simulink model "EVCS_model_v2"  (R2024b)
settings: Solver=VariableStepAuto  StartTime=0.0  StopTime=210  MaxStep=1e-3  RelTol=1e-2  AbsTol=1e-3
undefined symbols (not defined in the file or in its folder): FC, gcbh, Ion, Lithium, P, sps_rtmsupport, Ts
libraries: spsSeriesRLCBranchLib x40, spsIGBTDiodeLib x8, slpidlib x7, spsVoltageMeasurementLib x7, spsCurrentMeasurementLib x6, eeGeneralControl x4, spsMosfetLib x4, spsPWMGeneratorDCDCLib x3, spsAlphaBetaZerotodq0Lib x2, spsBatteryLib x2, spsDiodeLib x2, spsBreakerLib x1
(part 2 of 2)

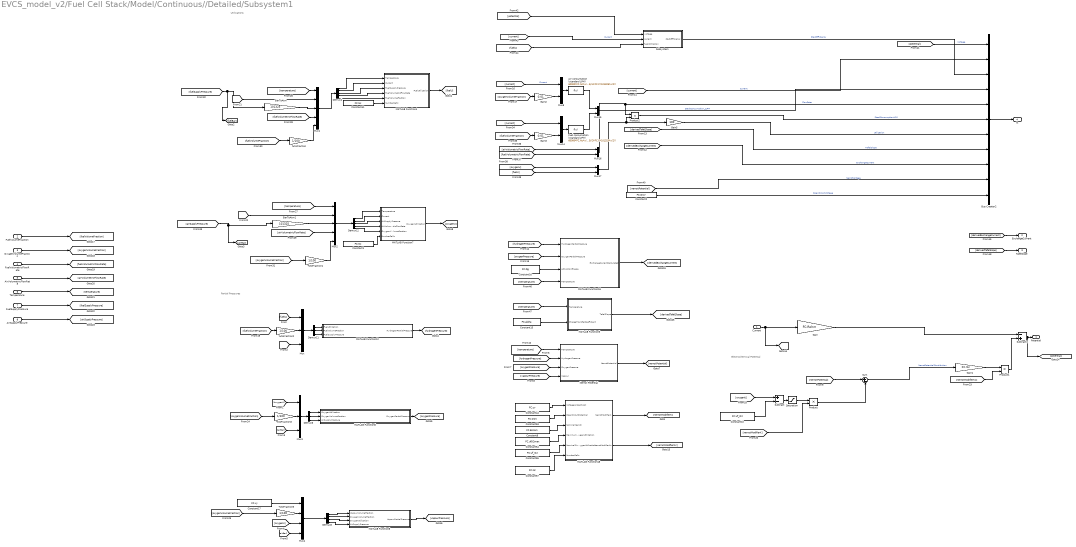
== system EVCS_model_v2/Fuel Cell Stack/Model/Continuous//Detailed/Subsystem1 ==
  note: Electrochemical Potential
  note: Partial Pressures
  note: Utilizations
  Current : Inport
  FuelVolumeFraction : Inport  Port=2
  OxygenVolumeFraction : Inport  Port=3
  FuelVolumetricFlowRate : Inport  Port=4
  AirVolumetricFlowRate : Inport  Port=5
  Temperature : Inport  Port=6
  FuelSupplyPressure : Inport  Port=7
  AirSupplyPressure : Inport  Port=8
  %toFraction{,1..3,5} (5 alike) : Gain  Gain=1/100
  Air consumption (standard LPM) : Fcn  Expr=60000*FC.Nc*u(1)*FC.R*293.15/(4*FC.F*101325*u(2))
  BarToAtm : Gain  Gain=101325
  BarToAtm1 : Gain  Gain=101325
  Bus Creator2 : BusCreator  Inputs=11
  Constant1 : Constant  Value=FC.Nc
  Constant10 : Constant  Value=FC.Uf_O2
  Constant15 : Constant  Value=FC.alpha
  Constant16 : Constant  Value=FC.Dg
  Constant17 : Constant  Value=FC.xy
  Constant2 : Constant  Value=FC.OCV
  Constant41 : Constant  Value=FC.Nc
  Constant44 : Constant  Value=FC.uv
  Constant53 : Constant  Value=FC.OCV
  Constant54 : Constant  Value=FC.ufO2max
  Constant55 : Constant  Value=FC.Uf_O2
  Constant57 : Constant  Value=FC.Nc
  Constant8 : Constant  Value=FC.Ennom
  Demux11 : Demux  Outputs=3
  Demux12 : Demux  Outputs=5
  Demux4 : Demux  Outputs=5
  Demux6 : Demux  Outputs=3
  Demux8 : Demux
  Fuel consumption (standard LPM) : Fcn  Expr=60000*FC.Nc*u(1)*FC.R*293.15/(2*FC.F*101325*u(2))
  Gain : Gain  Gain=FC.Rohm
  Gain1 : Gain  Gain=FC.Nc
  Gain2 : Gain  Gain=0.01
  Gain3 : Gain  Gain=0.01
  Gain5 : Gain  Gain=100
  MATLAB Function12 : MATLAB Function  TreatAsAtomicUnit=on
  MATLAB Function16 : MATLAB Function  TreatAsAtomicUnit=on
  MATLAB Function18 : MATLAB Function  TreatAsAtomicUnit=on
  MATLAB Function4 : MATLAB Function  TreatAsAtomicUnit=on
  MATLAB Function5 : MATLAB Function  TreatAsAtomicUnit=on
  MATLAB Function6 : MATLAB Function  TreatAsAtomicUnit=on
  MATLAB Function7 : MATLAB Function  TreatAsAtomicUnit=on
  MATLAB Function8 : MATLAB Function  TreatAsAtomicUnit=on
  Mux : Mux  Inputs=3
  Mux1 : Mux  Inputs=5
  Mux{8,14..17} (5 alike) : Mux  Inputs=2
  Mux2 : Mux  Inputs=5
  Mux3 : Mux  Inputs=3
  Mux4 : Mux
  Nernst Potential : Subsystem
  Product : Product
  Product1 : Product
  Product2 : Product  RndMeth=Zero
  Saturation : Saturate  UpperLimit=inf  LowerLimit=0
  Subsystem : Subsystem
  Subtract : Sum  Inputs=+-
  Subtract1 : Sum  Inputs=-+
  Sum : Sum  Inputs=|+-
  Potential : Outport
  ExchangeCurrent : Outport  Port=2
  TafelSlope : Outport  Port=3
  m : Outport  Port=4
  wires:
  %toFraction3/1 -> Mux3/2
  Constant2/1 -> Bus Creator2/11  "OpenCircuitVoltage"
  Demux4/4 -> MATLAB Function4/4(FuelVolumetricFlowRate)
  [temperature] -> MATLAB Function16/4(Temperature)
  [oxygenU] -> Mux3/1
  Demux4/1 -> MATLAB Function4/1(Temperature)
  AirSupplyPressure/1 -> [airSupplyPressure]
  [fuelVolumeFraction] -> Gain3/1
  BarToAtm1/1 -> Mux2/3
  Constant55/1 -> MATLAB Function18/5(NominalOxygenUtilization)
  [oxygenVolumeFraction] -> %toFraction5/1
  [airVolumetricFlowRate] -> Mux16/1
  Demux4/5 -> MATLAB Function4/5(FuelVolumeFraction)
  [oxygenU] -> Mux17/1
  Gain5/1 -> Bus Creator2/7  "Utilization"
  [fuelVolumeFraction] -> %toFraction2/1
  [potential] -> Subsystem/1(voltage)
  Mux17/1 -> Product2/2, Gain5/1
  Demux8/2 -> MATLAB Function8/2(OxygenVolumeFraction)
  Demux4/3 -> MATLAB Function4/3(FuelSupplyPressure)
  MATLAB Function7/1(OxygenUtilization) -> [oxygenU]
  [current] -> Mux1/2
  [nernstPotential] -> Bus Creator2/10  "NernstVoltage"
  Product1/1 -> Subtract1/2
  Demux11/3 -> MATLAB Function12/3(FuelSupplyPressure)
  Constant1/1 -> MATLAB Function7/6(NumberCells)
  AirVolumetricFlowRate/1 -> [airVolumetricFlowRate]
  [fuelVolumetricFlowRate] -> Mux16/2
  MATLAB Function8/1(VapourPartialPressure) -> [vapourPressure]
  Subtract1/1 -> [potential], Potential/1
  Bus Creator2/1 -> m/1
  [temperature] -> Nernst Potential/1(Temperature)
  %toFraction5/1 -> Mux4/2
  [fuelVolumetricFlowRate] -> Mux1/4
  Demux11/2 -> MATLAB Function12/2(FuelVolumeFraction)
  Demux8/1 -> MATLAB Function8/1(VapourVolumeFraction)
  Gain/1 -> Subtract1/1
  [oxygenVolumeFraction] -> %toFraction1/1
  [potential] -> Bus Creator2/1  "Voltage"
  Constant44/1 -> MATLAB Function18/1(VoltageUndershoot)
  Demux6/1 -> MATLAB Function6/1(OxygenUtilization)
  [fuelVolumeFraction] -> %toFraction/1
  Mux8/1 -> Air consumption (standard LPM)/1
  [oxygenU] -> Mux4/3
  [oxygenVolumeFraction] -> %toFraction3/1
  MATLAB Function16/1(ExchangeCurrentCalculated) -> [derivedExchangeCurrent]
  [temperature] -> Mux2/1
  [hydrogenPressure] -> MATLAB Function16/1(HydrogenPartialPressure)
  Subsystem/1(stackEfficiency) -> Bus Creator2/3  "StackEfficiency"
  Demux12/4 -> MATLAB Function7/4(AirVolumetricFlowRate)
  Demux12/2 -> MATLAB Function7/2(Current)
  MATLAB Function12/1(HydrogenPartialPressure) -> [hydrogenPressure]
  MATLAB Function18/1(NernstModifierK) -> [nernstModifierK]
  MATLAB Function5/1(TafelSlope) -> [derivedTafelSlope]
  Constant15/1 -> MATLAB Function5/2(ChargeTransferCoefficient)
  [fuelU] -> Mux17/2
  Mux14/1 -> Fuel consumption (standard LPM)/1
  FuelVolumeFraction/1 -> [fuelVolumeFraction]
  FuelVolumetricFlowRate/1 -> [fuelVolumetricFlowRate]
  [derivedExchangeCurrent] -> Bus Creator2/9  "ExchangeCurrent"
  FuelSupplyPressure/1 -> [fuelSupplyPressure]
  Demux12/1 -> MATLAB Function7/1(Temperature)
  Sum/1 -> Gain1/1  "NernstPotentialContribution"
  [airVolumetricFlowRate] -> Mux2/4
  Mux1/1 -> Demux4/1
  Product/1 -> Sum/2
  Fuel consumption (standard LPM)/1 -> Mux15/2
  Mux3/1 -> Demux6/1
  Product2/1 -> Bus Creator2/6  "StackConsumptionLPM"
  Saturation/1 -> Product/1
  [current] -> Mux2/2
  Mux15/1 -> Bus Creator2/4  "StackConsumption_sLPM"
  [current] -> Bus Creator2/2  "Current"
  Constant41/1 -> MATLAB Function4/6(NumberCells)
  %toFraction/1 -> Mux1/5
  OxygenVolumeFraction/1 -> [oxygenVolumeFraction]
  [airBar] -> Mux3/3
  Constant10/1 -> Subtract/2
  [fuelU] -> Mux/1
  [oxygenVolumeFraction] -> Gain2/1
  [oxygenPressure] -> Nernst Potential/3(OxygenPressure)
  Gain1/1 -> Product1/1
  [current] -> Subsystem/2(current)  "Current"
  Constant53/1 -> MATLAB Function18/2(OpenCircuitPotential)
  Demux11/1 -> MATLAB Function12/1(FuelUtilization)
  [nernstModifierKc] -> Product1/2
  Temperature/1 -> [temperature]
  [current] -> Mux14/1
  [airBar] -> Mux4/4
  Demux12/5 -> MATLAB Function7/5(OxygenVolumeFraction)
  Constant57/1 -> MATLAB Function18/6(NumberCells)
  Air consumption (standard LPM)/1 -> Mux15/1
  [nernstPotential] -> Sum/1
  [fuelSupplyPressure] -> BarToAtm/1, [fuelBar]
  [airSupplyPressure] -> BarToAtm1/1, [airBar]
  Nernst Potential/1(NernstPotential) -> [nernstPotential]
  [oxygenU] -> Subtract/1
  %toFraction1/1 -> Mux2/5
  [temperature] -> Mux1/1
  Demux12/3 -> MATLAB Function7/3(AirSupplyPressure)
  [hydrogenPressure] -> Nernst Potential/2(HydrogenPressure)
  Demux6/3 -> MATLAB Function6/3(AirSupplyPressure)
  Constant17/1 -> Mux4/1
  Mux16/1 -> Product2/1, Bus Creator2/5  "FlowRate"
  Demux8/3 -> MATLAB Function8/3(OxygenUtilization)
  MATLAB Function18/2(NernstModifierKc) -> [nernstModifierKc]
  Current/1 -> [current], Gain/1
  Mux2/1 -> Demux12/1
  BarToAtm/1 -> Mux1/3
  Constant8/1 -> MATLAB Function18/3(NominalNernst)
  [current] -> Mux8/1  "Current"
  [oxygenPressure] -> MATLAB Function16/2(OxygenPartialPressure)
  [fuelU] -> Subsystem/3(fuelUtilization)
  Demux6/2 -> MATLAB Function6/2(OxygenVolumeFraction)
  [derivedTafelSlope] -> TafelSlope/1
  MATLAB Function6/1(OxygenPartialPressure) -> [oxygenPressure]
  [vapourPressure] -> Nernst Potential/4(Vapour)
  Demux4/2 -> MATLAB Function4/2(Current)
  Gain2/1 -> Mux8/2
  Constant16/1 -> MATLAB Function16/3(ActivationEnergy)
  [fuelBar] -> Mux/3
  Mux4/1 -> Demux8/1
  [temperature] -> MATLAB Function5/1(Temperature)
  Subtract/1 -> Saturation/1
  [derivedExchangeCurrent] -> ExchangeCurrent/1
  [derivedTafelSlope] -> Bus Creator2/8  "TafelSlope"
  %toFraction2/1 -> Mux/2
  Gain3/1 -> Mux14/2
  MATLAB Function4/1(FuelUtilization) -> [fuelU]
  Demux8/4 -> MATLAB Function8/4(AirSupplyPressure)
  Constant54/1 -> MATLAB Function18/4(MaximumOxygenUtilization)
  [nernstModifierK] -> Product/2
  Mux/1 -> Demux11/1

== system EVCS_model_v2/Fuel Cell Stack/Model/Continuous//Simplified/Subsystem ==
  Current : Inport
  exchangeCurrent : Inport  Port=2
  tafelSlope : Inport  Port=3
  Constant : Constant  Value=1e-9
  Divide : Product  Inputs=*/
  Gain : Gain  Gain=FC.Nc
  Low-Pass Filter (Discrete or Continuous) : eeGeneralControl/Low-Pass Filter (Discrete or Continuous)  K=1  T=FC.Tau  B=inf  A=-inf  init_option=Specify as parameter  x0=0  Ts=Ts
  Math Function : Math  Operator=log
  Product : Product
  Saturation : Saturate  UpperLimit=inf  LowerLimit=0
  Sum : Sum  Inputs=++|
  delayedActivationOverpotential : Outport
  wires:
  Current/1 -> Sum/2
  Gain/1 -> Product/2
  Constant/1 -> Sum/1
  tafelSlope/1 -> Gain/1
  Saturation/1 -> delayedActivationOverpotential/1
  Product/1 -> Low-Pass Filter (Discrete or Continuous)/1
  Sum/1 -> Divide/1
  Divide/1 -> Math Function/1
  Math Function/1 -> Product/1
  Low-Pass Filter (Discrete or Continuous)/1 -> Saturation/1
  exchangeCurrent/1 -> Divide/2

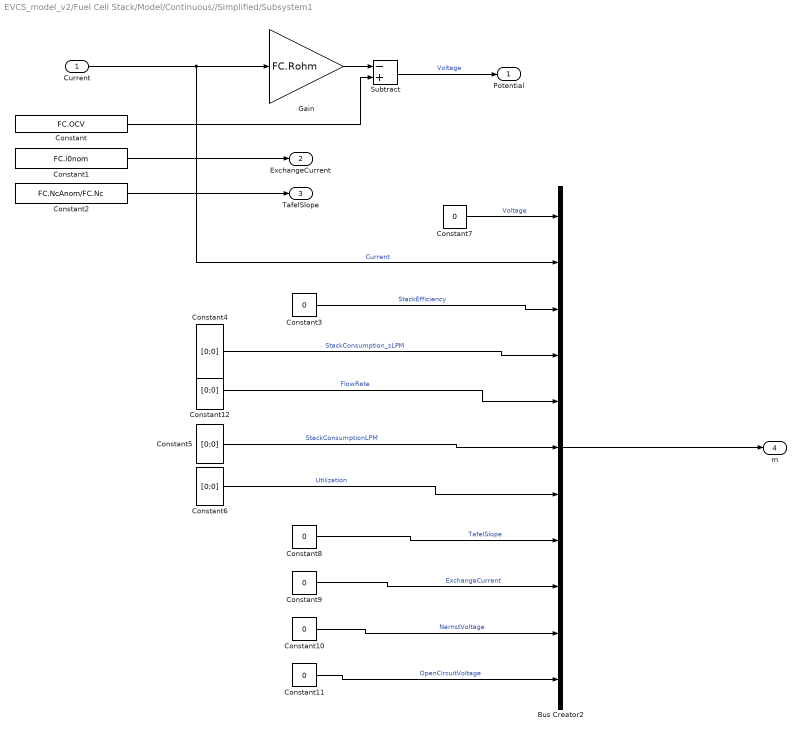
== system EVCS_model_v2/Fuel Cell Stack/Model/Continuous//Simplified/Subsystem1 ==
  Current : Inport
  Bus Creator2 : BusCreator  Inputs=11
  Constant : Constant  Value=FC.OCV
  Constant1 : Constant  Value=FC.i0nom
  Constant{3,7..11} (6 alike) : Constant  Value=0
  Constant{4..6,12} (4 alike) : Constant  Value=[0;0]
  Constant2 : Constant  Value=FC.NcAnom/FC.Nc
  Gain : Gain  Gain=FC.Rohm
  Subtract : Sum  Inputs=-+
  Potential : Outport
  ExchangeCurrent : Outport  Port=2
  TafelSlope : Outport  Port=3
  m : Outport  Port=4
  wires:
  Constant7/1 -> Bus Creator2/1  "Voltage"
  Constant12/1 -> Bus Creator2/5  "FlowRate"
  Constant8/1 -> Bus Creator2/8  "TafelSlope"
  Constant5/1 -> Bus Creator2/6  "StackConsumptionLPM"
  Bus Creator2/1 -> m/1
  Subtract/1 -> Potential/1  "Voltage"
  Gain/1 -> Subtract/1
  Constant2/1 -> TafelSlope/1
  Constant/1 -> Subtract/2
  Constant6/1 -> Bus Creator2/7  "Utilization"
  Constant9/1 -> Bus Creator2/9  "ExchangeCurrent"
  Constant1/1 -> ExchangeCurrent/1
  Constant11/1 -> Bus Creator2/11  "OpenCircuitVoltage"
  Constant3/1 -> Bus Creator2/3  "StackEfficiency"
  Constant10/1 -> Bus Creator2/10  "NernstVoltage"
  Constant4/1 -> Bus Creator2/4  "StackConsumption_sLPM"
  Current/1 -> Gain/1, Bus Creator2/2  "Current"

== system EVCS_model_v2/Fuel Cell Stack/Model/Discrete//Detailed/Subsystem ==
  Current : Inport
  exchangeCurrent : Inport  Port=2
  tafelSlope : Inport  Port=3
  Constant : Constant  Value=1e-9
  Divide : Product  Inputs=*/
  Gain : Gain  Gain=FC.Nc
  Low-Pass Filter (Discrete or Continuous) : eeGeneralControl/Low-Pass Filter (Discrete or Continuous)  K=1  T=FC.Tau  B=inf  A=-inf  init_option=Specify as parameter  x0=0  Ts=Ts
  Math Function : Math  Operator=log
  Product : Product
  Saturation : Saturate  UpperLimit=inf  LowerLimit=0
  Sum : Sum  Inputs=++|
  delayedActivationOverpotential : Outport
  wires:
  Current/1 -> Sum/2
  Gain/1 -> Product/2
  Constant/1 -> Sum/1
  tafelSlope/1 -> Gain/1
  Saturation/1 -> delayedActivationOverpotential/1
  Product/1 -> Low-Pass Filter (Discrete or Continuous)/1
  Sum/1 -> Divide/1
  Divide/1 -> Math Function/1
  Math Function/1 -> Product/1
  Low-Pass Filter (Discrete or Continuous)/1 -> Saturation/1
  exchangeCurrent/1 -> Divide/2

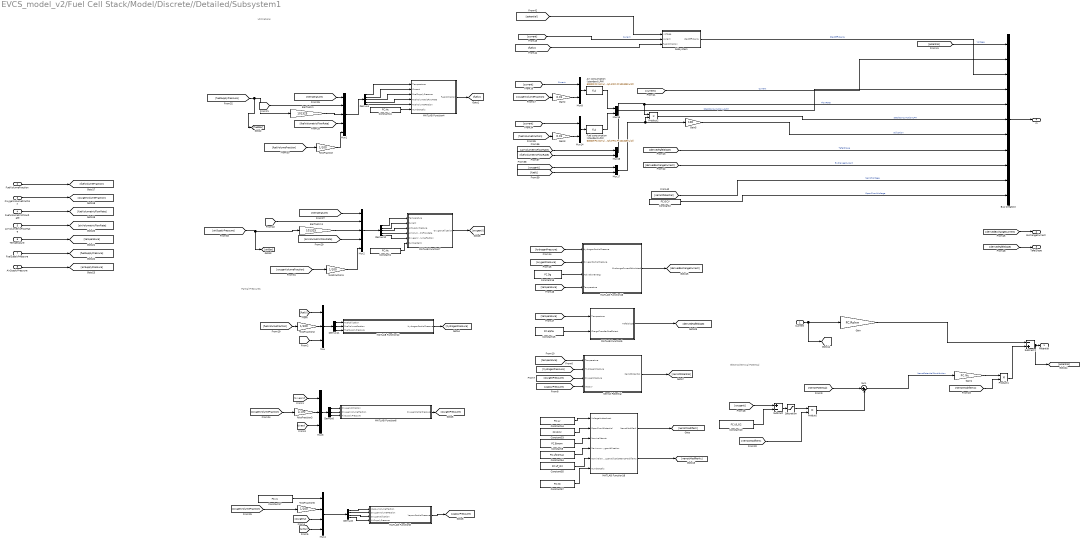
== system EVCS_model_v2/Fuel Cell Stack/Model/Discrete//Detailed/Subsystem1 ==
  note: Electrochemical Potential
  note: Partial Pressures
  note: Utilizations
  Current : Inport
  FuelVolumeFraction : Inport  Port=2
  OxygenVolumeFraction : Inport  Port=3
  FuelVolumetricFlowRate : Inport  Port=4
  AirVolumetricFlowRate : Inport  Port=5
  Temperature : Inport  Port=6
  FuelSupplyPressure : Inport  Port=7
  AirSupplyPressure : Inport  Port=8
  %toFraction{,1..3,5} (5 alike) : Gain  Gain=1/100
  Air consumption (standard LPM) : Fcn  Expr=60000*FC.Nc*u(1)*FC.R*293.15/(4*FC.F*101325*u(2))
  BarToAtm : Gain  Gain=101325
  BarToAtm1 : Gain  Gain=101325
  Bus Creator2 : BusCreator  Inputs=11
  Constant1 : Constant  Value=FC.Nc
  Constant10 : Constant  Value=FC.Uf_O2
  Constant15 : Constant  Value=FC.alpha
  Constant16 : Constant  Value=FC.Dg
  Constant17 : Constant  Value=FC.xy
  Constant2 : Constant  Value=FC.OCV
  Constant41 : Constant  Value=FC.Nc
  Constant44 : Constant  Value=FC.uv
  Constant53 : Constant  Value=FC.OCV
  Constant54 : Constant  Value=FC.ufO2max
  Constant55 : Constant  Value=FC.Uf_O2
  Constant57 : Constant  Value=FC.Nc
  Constant8 : Constant  Value=FC.Ennom
  Demux11 : Demux  Outputs=3
  Demux12 : Demux  Outputs=5
  Demux4 : Demux  Outputs=5
  Demux6 : Demux  Outputs=3
  Demux8 : Demux
  Fuel consumption (standard LPM) : Fcn  Expr=60000*FC.Nc*u(1)*FC.R*293.15/(2*FC.F*101325*u(2))
  Gain : Gain  Gain=FC.Rohm
  Gain1 : Gain  Gain=FC.Nc
  Gain2 : Gain  Gain=0.01
  Gain3 : Gain  Gain=0.01
  Gain5 : Gain  Gain=100
  MATLAB Function12 : MATLAB Function  TreatAsAtomicUnit=on
  MATLAB Function16 : MATLAB Function  TreatAsAtomicUnit=on
  MATLAB Function18 : MATLAB Function  TreatAsAtomicUnit=on
  MATLAB Function4 : MATLAB Function  TreatAsAtomicUnit=on
  MATLAB Function5 : MATLAB Function  TreatAsAtomicUnit=on
  MATLAB Function6 : MATLAB Function  TreatAsAtomicUnit=on
  MATLAB Function7 : MATLAB Function  TreatAsAtomicUnit=on
  MATLAB Function8 : MATLAB Function  TreatAsAtomicUnit=on
  Mux : Mux  Inputs=3
  Mux1 : Mux  Inputs=5
  Mux{8,14..17} (5 alike) : Mux  Inputs=2
  Mux2 : Mux  Inputs=5
  Mux3 : Mux  Inputs=3
  Mux4 : Mux
  Nernst Potential : Subsystem
  Product : Product
  Product1 : Product
  Product2 : Product  RndMeth=Zero
  Saturation : Saturate  UpperLimit=inf  LowerLimit=0
  Subsystem : Subsystem
  Subtract : Sum  Inputs=+-
  Subtract1 : Sum  Inputs=-+
  Sum : Sum  Inputs=|+-
  Potential : Outport
  ExchangeCurrent : Outport  Port=2
  TafelSlope : Outport  Port=3
  m : Outport  Port=4
  wires:
  %toFraction3/1 -> Mux3/2
  Constant2/1 -> Bus Creator2/11  "OpenCircuitVoltage"
  Demux4/4 -> MATLAB Function4/4(FuelVolumetricFlowRate)
  [temperature] -> MATLAB Function16/4(Temperature)
  [oxygenU] -> Mux3/1
  Demux4/1 -> MATLAB Function4/1(Temperature)
  AirSupplyPressure/1 -> [airSupplyPressure]
  [fuelVolumeFraction] -> Gain3/1
  BarToAtm1/1 -> Mux2/3
  Constant55/1 -> MATLAB Function18/5(NominalOxygenUtilization)
  [oxygenVolumeFraction] -> %toFraction5/1
  [airVolumetricFlowRate] -> Mux16/1
  Demux4/5 -> MATLAB Function4/5(FuelVolumeFraction)
  [oxygenU] -> Mux17/1
  Gain5/1 -> Bus Creator2/7  "Utilization"
  [fuelVolumeFraction] -> %toFraction2/1
  [potential] -> Subsystem/1(voltage)
  Mux17/1 -> Product2/2, Gain5/1
  Demux8/2 -> MATLAB Function8/2(OxygenVolumeFraction)
  Demux4/3 -> MATLAB Function4/3(FuelSupplyPressure)
  MATLAB Function7/1(OxygenUtilization) -> [oxygenU]
  [current] -> Mux1/2
  [nernstPotential] -> Bus Creator2/10  "NernstVoltage"
  Product1/1 -> Subtract1/2
  Demux11/3 -> MATLAB Function12/3(FuelSupplyPressure)
  Constant1/1 -> MATLAB Function7/6(NumberCells)
  AirVolumetricFlowRate/1 -> [airVolumetricFlowRate]
  [fuelVolumetricFlowRate] -> Mux16/2
  MATLAB Function8/1(VapourPartialPressure) -> [vapourPressure]
  Subtract1/1 -> [potential], Potential/1
  Bus Creator2/1 -> m/1
  [temperature] -> Nernst Potential/1(Temperature)
  %toFraction5/1 -> Mux4/2
  [fuelVolumetricFlowRate] -> Mux1/4
  Demux11/2 -> MATLAB Function12/2(FuelVolumeFraction)
  Demux8/1 -> MATLAB Function8/1(VapourVolumeFraction)
  Gain/1 -> Subtract1/1
  [oxygenVolumeFraction] -> %toFraction1/1
  [potential] -> Bus Creator2/1  "Voltage"
  Constant44/1 -> MATLAB Function18/1(VoltageUndershoot)
  Demux6/1 -> MATLAB Function6/1(OxygenUtilization)
  [fuelVolumeFraction] -> %toFraction/1
  Mux8/1 -> Air consumption (standard LPM)/1
  [oxygenU] -> Mux4/3
  [oxygenVolumeFraction] -> %toFraction3/1
  MATLAB Function16/1(ExchangeCurrentCalculated) -> [derivedExchangeCurrent]
  [temperature] -> Mux2/1
  [hydrogenPressure] -> MATLAB Function16/1(HydrogenPartialPressure)
  Subsystem/1(stackEfficiency) -> Bus Creator2/3  "StackEfficiency"
  Demux12/4 -> MATLAB Function7/4(AirVolumetricFlowRate)
  Demux12/2 -> MATLAB Function7/2(Current)
  MATLAB Function12/1(HydrogenPartialPressure) -> [hydrogenPressure]
  MATLAB Function18/1(NernstModifierK) -> [nernstModifierK]
  MATLAB Function5/1(TafelSlope) -> [derivedTafelSlope]
  Constant15/1 -> MATLAB Function5/2(ChargeTransferCoefficient)
  [fuelU] -> Mux17/2
  Mux14/1 -> Fuel consumption (standard LPM)/1
  FuelVolumeFraction/1 -> [fuelVolumeFraction]
  FuelVolumetricFlowRate/1 -> [fuelVolumetricFlowRate]
  [derivedExchangeCurrent] -> Bus Creator2/9  "ExchangeCurrent"
  FuelSupplyPressure/1 -> [fuelSupplyPressure]
  Demux12/1 -> MATLAB Function7/1(Temperature)
  Sum/1 -> Gain1/1  "NernstPotentialContribution"
  [airVolumetricFlowRate] -> Mux2/4
  Mux1/1 -> Demux4/1
  Product/1 -> Sum/2
  Fuel consumption (standard LPM)/1 -> Mux15/2
  Mux3/1 -> Demux6/1
  Product2/1 -> Bus Creator2/6  "StackConsumptionLPM"
  Saturation/1 -> Product/1
  [current] -> Mux2/2
  Mux15/1 -> Bus Creator2/4  "StackConsumption_sLPM"
  [current] -> Bus Creator2/2  "Current"
  Constant41/1 -> MATLAB Function4/6(NumberCells)
  %toFraction/1 -> Mux1/5
  OxygenVolumeFraction/1 -> [oxygenVolumeFraction]
  [airBar] -> Mux3/3
  Constant10/1 -> Subtract/2
  [fuelU] -> Mux/1
  [oxygenVolumeFraction] -> Gain2/1
  [oxygenPressure] -> Nernst Potential/3(OxygenPressure)
  Gain1/1 -> Product1/1
  [current] -> Subsystem/2(current)  "Current"
  Constant53/1 -> MATLAB Function18/2(OpenCircuitPotential)
  Demux11/1 -> MATLAB Function12/1(FuelUtilization)
  [nernstModifierKc] -> Product1/2
  Temperature/1 -> [temperature]
  [current] -> Mux14/1
  [airBar] -> Mux4/4
  Demux12/5 -> MATLAB Function7/5(OxygenVolumeFraction)
  Constant57/1 -> MATLAB Function18/6(NumberCells)
  Air consumption (standard LPM)/1 -> Mux15/1
  [nernstPotential] -> Sum/1
  [fuelSupplyPressure] -> BarToAtm/1, [fuelBar]
  [airSupplyPressure] -> BarToAtm1/1, [airBar]
  Nernst Potential/1(NernstPotential) -> [nernstPotential]
  [oxygenU] -> Subtract/1
  %toFraction1/1 -> Mux2/5
  [temperature] -> Mux1/1
  Demux12/3 -> MATLAB Function7/3(AirSupplyPressure)
  [hydrogenPressure] -> Nernst Potential/2(HydrogenPressure)
  Demux6/3 -> MATLAB Function6/3(AirSupplyPressure)
  Constant17/1 -> Mux4/1
  Mux16/1 -> Product2/1, Bus Creator2/5  "FlowRate"
  Demux8/3 -> MATLAB Function8/3(OxygenUtilization)
  MATLAB Function18/2(NernstModifierKc) -> [nernstModifierKc]
  Current/1 -> [current], Gain/1
  Mux2/1 -> Demux12/1
  BarToAtm/1 -> Mux1/3
  Constant8/1 -> MATLAB Function18/3(NominalNernst)
  [current] -> Mux8/1  "Current"
  [oxygenPressure] -> MATLAB Function16/2(OxygenPartialPressure)
  [fuelU] -> Subsystem/3(fuelUtilization)
  Demux6/2 -> MATLAB Function6/2(OxygenVolumeFraction)
  [derivedTafelSlope] -> TafelSlope/1
  MATLAB Function6/1(OxygenPartialPressure) -> [oxygenPressure]
  [vapourPressure] -> Nernst Potential/4(Vapour)
  Demux4/2 -> MATLAB Function4/2(Current)
  Gain2/1 -> Mux8/2
  Constant16/1 -> MATLAB Function16/3(ActivationEnergy)
  [fuelBar] -> Mux/3
  Mux4/1 -> Demux8/1
  [temperature] -> MATLAB Function5/1(Temperature)
  Subtract/1 -> Saturation/1
  [derivedExchangeCurrent] -> ExchangeCurrent/1
  [derivedTafelSlope] -> Bus Creator2/8  "TafelSlope"
  %toFraction2/1 -> Mux/2
  Gain3/1 -> Mux14/2
  MATLAB Function4/1(FuelUtilization) -> [fuelU]
  Demux8/4 -> MATLAB Function8/4(AirSupplyPressure)
  Constant54/1 -> MATLAB Function18/4(MaximumOxygenUtilization)
  [nernstModifierK] -> Product/2
  Mux/1 -> Demux11/1

== system EVCS_model_v2/Fuel Cell Stack/Model/Discrete//Simplified/Subsystem ==
  Current : Inport
  exchangeCurrent : Inport  Port=2
  tafelSlope : Inport  Port=3
  Constant : Constant  Value=1e-9
  Divide : Product  Inputs=*/
  Gain : Gain  Gain=FC.Nc
  Low-Pass Filter (Discrete or Continuous) : eeGeneralControl/Low-Pass Filter (Discrete or Continuous)  K=1  T=FC.Tau  B=inf  A=-inf  init_option=Specify as parameter  x0=0  Ts=Ts
  Math Function : Math  Operator=log
  Product : Product
  Saturation : Saturate  UpperLimit=inf  LowerLimit=0
  Sum : Sum  Inputs=++|
  delayedActivationOverpotential : Outport
  wires:
  Current/1 -> Sum/2
  Gain/1 -> Product/2
  Constant/1 -> Sum/1
  tafelSlope/1 -> Gain/1
  Saturation/1 -> delayedActivationOverpotential/1
  Product/1 -> Low-Pass Filter (Discrete or Continuous)/1
  Sum/1 -> Divide/1
  Divide/1 -> Math Function/1
  Math Function/1 -> Product/1
  Low-Pass Filter (Discrete or Continuous)/1 -> Saturation/1
  exchangeCurrent/1 -> Divide/2

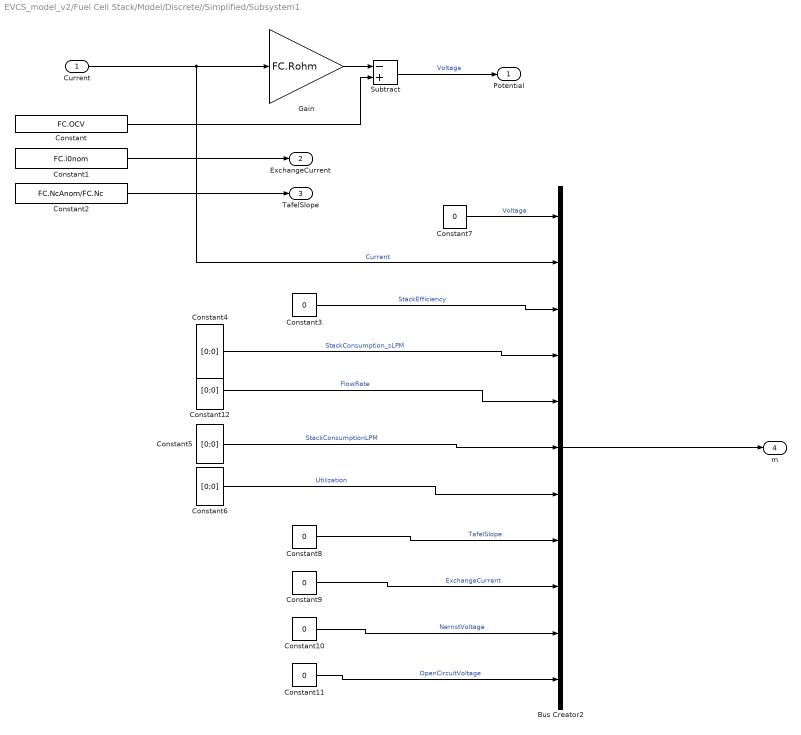
== system EVCS_model_v2/Fuel Cell Stack/Model/Discrete//Simplified/Subsystem1 ==
  Current : Inport
  Bus Creator2 : BusCreator  Inputs=11
  Constant : Constant  Value=FC.OCV
  Constant1 : Constant  Value=FC.i0nom
  Constant{3,7..11} (6 alike) : Constant  Value=0
  Constant{4..6,12} (4 alike) : Constant  Value=[0;0]
  Constant2 : Constant  Value=FC.NcAnom/FC.Nc
  Gain : Gain  Gain=FC.Rohm
  Subtract : Sum  Inputs=-+
  Potential : Outport
  ExchangeCurrent : Outport  Port=2
  TafelSlope : Outport  Port=3
  m : Outport  Port=4
  wires:
  Constant7/1 -> Bus Creator2/1  "Voltage"
  Constant12/1 -> Bus Creator2/5  "FlowRate"
  Constant8/1 -> Bus Creator2/8  "TafelSlope"
  Constant5/1 -> Bus Creator2/6  "StackConsumptionLPM"
  Bus Creator2/1 -> m/1
  Subtract/1 -> Potential/1  "Voltage"
  Gain/1 -> Subtract/1
  Constant2/1 -> TafelSlope/1
  Constant/1 -> Subtract/2
  Constant6/1 -> Bus Creator2/7  "Utilization"
  Constant9/1 -> Bus Creator2/9  "ExchangeCurrent"
  Constant1/1 -> ExchangeCurrent/1
  Constant11/1 -> Bus Creator2/11  "OpenCircuitVoltage"
  Constant3/1 -> Bus Creator2/3  "StackEfficiency"
  Constant10/1 -> Bus Creator2/10  "NernstVoltage"
  Constant4/1 -> Bus Creator2/4  "StackConsumption_sLPM"
  Current/1 -> Gain/1, Bus Creator2/2  "Current"

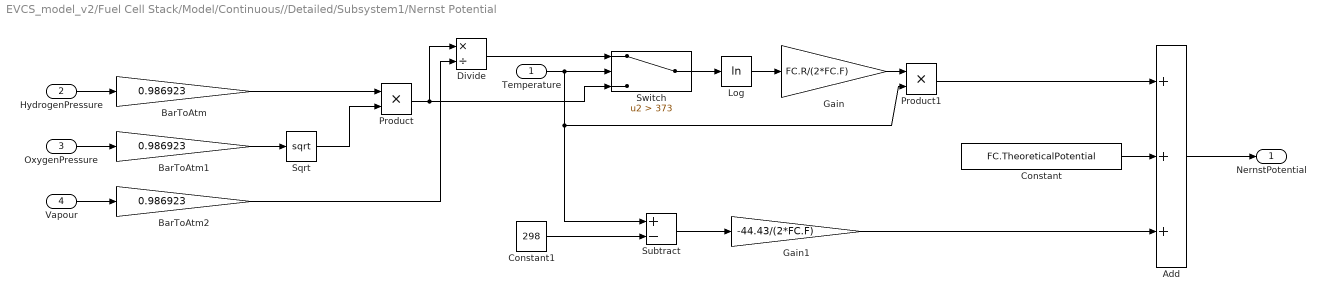
== system EVCS_model_v2/Fuel Cell Stack/Model/Continuous//Detailed/Subsystem1/Nernst Potential ==
  Temperature : Inport
  HydrogenPressure : Inport  Port=2
  OxygenPressure : Inport  Port=3
  Vapour : Inport  Port=4
  Add : Sum  Inputs=+++
  BarToAtm : Gain  Gain=0.986923
  BarToAtm1 : Gain  Gain=0.986923
  BarToAtm2 : Gain  Gain=0.986923
  Constant : Constant  Value=FC.TheoreticalPotential
  Constant1 : Constant  Value=298
  Divide : Product  Inputs=*/
  Gain : Gain  Gain=FC.R/(2*FC.F)
  Gain1 : Gain  Gain=-44.43/(2*FC.F)
  Log : Math  Operator=log
  Product : Product
  Product1 : Product
  Sqrt : Sqrt
  Subtract : Sum  Inputs=+-
  Switch : Switch  Criteria=u2 > Threshold  Threshold=373  SaturateOnIntegerOverflow=off  InputSameDT=off
  NernstPotential : Outport
  wires:
  Add/1 -> NernstPotential/1
  Temperature/1 -> Product1/2, Subtract/1, Switch/2
  HydrogenPressure/1 -> BarToAtm/1
  OxygenPressure/1 -> BarToAtm1/1
  Vapour/1 -> BarToAtm2/1
  BarToAtm1/1 -> Sqrt/1
  Switch/1 -> Log/1
  Product/1 -> Divide/1, Switch/3
  Sqrt/1 -> Product/2
  BarToAtm/1 -> Product/1
  Divide/1 -> Switch/1
  BarToAtm2/1 -> Divide/2
  Log/1 -> Gain/1
  Gain/1 -> Product1/1
  Product1/1 -> Add/1
  Constant/1 -> Add/2
  Constant1/1 -> Subtract/2
  Subtract/1 -> Gain1/1
  Gain1/1 -> Add/3

== system EVCS_model_v2/Fuel Cell Stack/Model/Continuous//Detailed/Subsystem1/Subsystem ==
  voltage : Inport
  current : Inport  Port=2
  fuelUtilization : Inport  Port=3
  " " : Saturate  UpperLimit=inf  LowerLimit=1e-6  LinearizeAsGain=off
  Add : Sum
  Constant : Constant  Value=1e-5
  Fcn2 : Fcn  Expr=u(1)-FC.Rohm*u(2)
  Fcn3 : Fcn  Expr=(FC.Dh0)*(FC.Nc*u(1))/(2*FC.F*u(2))
  Gain6 : Gain  Gain=100
  Mux18 : Mux  Inputs=2
  Mux19 : Mux  Inputs=2
  Product3 : Product  RndMeth=Zero
  Product4 : Product  Inputs=*/  RndMeth=Zero
  zero avoider2 : Saturate  UpperLimit=inf  LowerLimit=0  LinearizeAsGain=off
  stackEfficiency : Outport
  wires:
  voltage/1 -> Mux18/1
  Gain6/1 -> stackEfficiency/1
  Fcn3/1 -> " "/1
  current/1 -> Product3/2, Mux18/2, Mux19/1
  fuelUtilization/1 -> Add/1
  Product3/1 -> zero avoider2/1
  Mux18/1 -> Fcn2/1
  Fcn2/1 -> Product3/1
  Mux19/1 -> Fcn3/1
  zero avoider2/1 -> Product4/1
  " "/1 -> Product4/2
  Product4/1 -> Gain6/1
  Add/1 -> Mux19/2
  Constant/1 -> Add/2

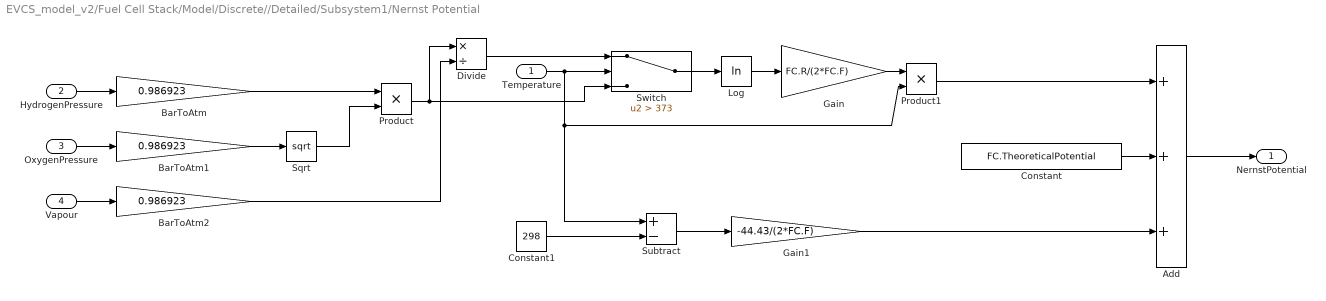
== system EVCS_model_v2/Fuel Cell Stack/Model/Discrete//Detailed/Subsystem1/Nernst Potential ==
  Temperature : Inport
  HydrogenPressure : Inport  Port=2
  OxygenPressure : Inport  Port=3
  Vapour : Inport  Port=4
  Add : Sum  Inputs=+++
  BarToAtm : Gain  Gain=0.986923
  BarToAtm1 : Gain  Gain=0.986923
  BarToAtm2 : Gain  Gain=0.986923
  Constant : Constant  Value=FC.TheoreticalPotential
  Constant1 : Constant  Value=298
  Divide : Product  Inputs=*/
  Gain : Gain  Gain=FC.R/(2*FC.F)
  Gain1 : Gain  Gain=-44.43/(2*FC.F)
  Log : Math  Operator=log
  Product : Product
  Product1 : Product
  Sqrt : Sqrt
  Subtract : Sum  Inputs=+-
  Switch : Switch  Criteria=u2 > Threshold  Threshold=373  SaturateOnIntegerOverflow=off  InputSameDT=off
  NernstPotential : Outport
  wires:
  Add/1 -> NernstPotential/1
  Temperature/1 -> Product1/2, Subtract/1, Switch/2
  HydrogenPressure/1 -> BarToAtm/1
  OxygenPressure/1 -> BarToAtm1/1
  Vapour/1 -> BarToAtm2/1
  BarToAtm1/1 -> Sqrt/1
  Switch/1 -> Log/1
  Product/1 -> Divide/1, Switch/3
  Sqrt/1 -> Product/2
  BarToAtm/1 -> Product/1
  Divide/1 -> Switch/1
  BarToAtm2/1 -> Divide/2
  Log/1 -> Gain/1
  Gain/1 -> Product1/1
  Product1/1 -> Add/1
  Constant/1 -> Add/2
  Constant1/1 -> Subtract/2
  Subtract/1 -> Gain1/1
  Gain1/1 -> Add/3

== system EVCS_model_v2/Fuel Cell Stack/Model/Discrete//Detailed/Subsystem1/Subsystem ==
  voltage : Inport
  current : Inport  Port=2
  fuelUtilization : Inport  Port=3
  " " : Saturate  UpperLimit=inf  LowerLimit=1e-6  LinearizeAsGain=off
  Add : Sum
  Constant : Constant  Value=1e-5
  Fcn2 : Fcn  Expr=u(1)-FC.Rohm*u(2)
  Fcn3 : Fcn  Expr=(FC.Dh0)*(FC.Nc*u(1))/(2*FC.F*u(2))
  Gain6 : Gain  Gain=100
  Mux18 : Mux  Inputs=2
  Mux19 : Mux  Inputs=2
  Product3 : Product  RndMeth=Zero
  Product4 : Product  Inputs=*/  RndMeth=Zero
  zero avoider2 : Saturate  UpperLimit=inf  LowerLimit=0  LinearizeAsGain=off
  stackEfficiency : Outport
  wires:
  voltage/1 -> Mux18/1
  Gain6/1 -> stackEfficiency/1
  Fcn3/1 -> " "/1
  current/1 -> Product3/2, Mux18/2, Mux19/1
  fuelUtilization/1 -> Add/1
  Product3/1 -> zero avoider2/1
  Mux18/1 -> Fcn2/1
  Fcn2/1 -> Product3/1
  Mux19/1 -> Fcn3/1
  zero avoider2/1 -> Product4/1
  " "/1 -> Product4/2
  Product4/1 -> Gain6/1
  Add/1 -> Mux19/2
  Constant/1 -> Add/2

== matlab function EVCS_model_v2/Fuel Cell Stack/Model/Continuous//Detailed/Subsystem1/MATLAB Function7 ==
  data: Temperature input; OxygenUtilization output; Current input; AirSupplyPressure input; AirVolumetricFlowRate input; OxygenVolumeFraction input; NumberCells input
function OxygenUtilization = calculateOxygenUtilization(Temperature, Current, AirSupplyPressure, AirVolumetricFlowRate, OxygenVolumeFraction, NumberCells)
    % Function to calculate oxygen utilization based on the given formula
    % Copyright 2024 The MathWorks, Inc.
    
    % Constants
    NumberElectrons = 4;
    OxygenUtilization = calculateUtilization(Temperature, Current, AirSupplyPressure, AirVolumetricFlowRate, OxygenVolumeFraction, NumberElectrons, NumberCells);
end

== matlab function EVCS_model_v2/Fuel Cell Stack/Model/Continuous//Detailed/Subsystem1/MATLAB Function8 ==
  data: VapourVolumeFraction input; OxygenVolumeFraction input; OxygenUtilization input; VapourPartialPressure output; AirSupplyPressure input
function VapourPartialPressure = calculateVapourPartialPressure(VapourVolumeFraction, OxygenVolumeFraction, OxygenUtilization, AirSupplyPressure)
    % Function to calculate vapour partial pressure
    
    % Copyright 2024 The MathWorks, Inc.
    
    VapourPartialPressure = calculateVapourPartialPressure(VapourVolumeFraction, OxygenVolumeFraction, OxygenUtilization, AirSupplyPressure);
end

== matlab function EVCS_model_v2/Fuel Cell Stack/Model/Discrete//Detailed/Subsystem1/MATLAB Function12 ==
  data: FuelUtilization input; HydrogenPartialPressure output; FuelVolumeFraction input; FuelSupplyPressure input
function HydrogenPartialPressure = calculateHydrogenPartialPressure(FuelUtilization, FuelVolumeFraction, FuelSupplyPressure)
    % Function to calculate hydrogen partial pressure
    % Copyright 2024 The MathWorks, Inc.
    
    HydrogenPartialPressure = calculatePartialPressure(FuelUtilization, FuelVolumeFraction, FuelSupplyPressure);
end

== matlab function EVCS_model_v2/Fuel Cell Stack/Model/Discrete//Detailed/Subsystem1/MATLAB Function16 ==
  data: HydrogenPartialPressure input; ExchangeCurrentCalculated output; OxygenPartialPressure input; ActivationEnergy input; Temperature input
function ExchangeCurrentCalculated= calculateExchangeCurrent(HydrogenPartialPressure,OxygenPartialPressure,ActivationEnergy,Temperature)
    % Function to calculate Exchange Current Derived
    % Copyright 2024 The MathWorks, Inc.    
    
    F = 96485; % Faraday constant : (A*s/mol)
    k = 1.38e-23; % Boltzmann's constant : (J/K)
    R = 8.3145; % Ideal gas constant : (J/mol*K)
    h = 6.626e-34; % Planck's constant : (J*s)

    ExchangeCurrentCalculated = (2*F*k*(1e5)*(HydrogenPartialPressure + OxygenPartialPressure)/(R*h))*exp(-ActivationEnergy/(R*Temperature));
end

== matlab function EVCS_model_v2/Fuel Cell Stack/Model/Discrete//Detailed/Subsystem1/MATLAB Function18 ==
  data: VoltageUndershoot input; NernstModifierK output; OpenCircuitPotential input; NominalNernst input; MaximumOxygenUtilization input; NominalOxygenUtilization input; NernstModifierKc output; NumberCells input
function [NernstModifierK, NernstModifierKc] = calculateNernstModifiers(VoltageUndershoot, OpenCircuitPotential, NominalNernst, MaximumOxygenUtilization, NominalOxygenUtilization, NumberCells)
    
% Copyright 2024 The MathWorks, Inc.

    [NernstModifierK, NernstModifierKc] = calculateNernstModifiers(VoltageUndershoot, OpenCircuitPotential, NominalNernst, MaximumOxygenUtilization, NominalOxygenUtilization, NumberCells);

end

== matlab function EVCS_model_v2/Fuel Cell Stack/Model/Discrete//Detailed/Subsystem1/MATLAB Function4 ==
  data: Temperature input; FuelUtilization output; Current input; FuelSupplyPressure input; FuelVolumetricFlowRate input; FuelVolumeFraction input; NumberCells input
function FuelUtilization = calculateFuelUtilization(Temperature, Current, FuelSupplyPressure, FuelVolumetricFlowRate, FuelVolumeFraction, NumberCells)
    % Function to calculate oxygen utilization based on the given formula
    % Copyright 2024 The MathWorks, Inc.

    % Constants
    NumberElectrons = 2;
    FuelUtilization = calculateUtilization(Temperature, Current, FuelSupplyPressure, FuelVolumetricFlowRate, FuelVolumeFraction, NumberElectrons, NumberCells);
end

== matlab function EVCS_model_v2/Fuel Cell Stack/Model/Discrete//Detailed/Subsystem1/MATLAB Function5 ==
  data: Temperature input; TafelSlope output; ChargeTransferCoefficient input
function TafelSlope = calculateTafelSlope(Temperature,ChargeTransferCoefficient)

    % Inputs
    % Temperature : (K)
    % ChargeTransferCoefficient : (1)
    % Output
    % ActivationEnergyBarrier : (J)
    % Constants
    F = 96485.33212; % Faraday's constant (C/mol)
    R = 8.3144621; % Universal gas constant (J/(mol*K))
    NumberElectrons = 2;

    % Calculation
    TafelSlope = (R*Temperature)/(NumberElectrons*ChargeTransferCoefficient*F);

== matlab function EVCS_model_v2/Fuel Cell Stack/Model/Discrete//Detailed/Subsystem1/MATLAB Function6 ==
  data: OxygenUtilization input; OxygenPartialPressure output; OxygenVolumeFraction input; AirSupplyPressure input
function OxygenPartialPressure = calculateOxygenPartialPressure(OxygenUtilization, OxygenVolumeFraction, AirSupplyPressure)
    % Function to calculate hydrogen partial pressure
    % Copyright 2024 The MathWorks, Inc.
    
    OxygenPartialPressure = calculatePartialPressure(OxygenUtilization, OxygenVolumeFraction, AirSupplyPressure);
end

== matlab function EVCS_model_v2/Fuel Cell Stack/Model/Discrete//Detailed/Subsystem1/MATLAB Function7 ==
  data: Temperature input; OxygenUtilization output; Current input; AirSupplyPressure input; AirVolumetricFlowRate input; OxygenVolumeFraction input; NumberCells input
function OxygenUtilization = calculateOxygenUtilization(Temperature, Current, AirSupplyPressure, AirVolumetricFlowRate, OxygenVolumeFraction, NumberCells)
    % Function to calculate oxygen utilization based on the given formula
    % Copyright 2024 The MathWorks, Inc.
    
    % Constants
    NumberElectrons = 4;
    OxygenUtilization = calculateUtilization(Temperature, Current, AirSupplyPressure, AirVolumetricFlowRate, OxygenVolumeFraction, NumberElectrons, NumberCells);
end

== matlab function EVCS_model_v2/Fuel Cell Stack/Model/Discrete//Detailed/Subsystem1/MATLAB Function8 ==
  data: VapourVolumeFraction input; OxygenVolumeFraction input; OxygenUtilization input; VapourPartialPressure output; AirSupplyPressure input
function VapourPartialPressure = calculateVapourPartialPressure(VapourVolumeFraction, OxygenVolumeFraction, OxygenUtilization, AirSupplyPressure)
    % Function to calculate vapour partial pressure
    
    % Copyright 2024 The MathWorks, Inc.
    
    VapourPartialPressure = calculateVapourPartialPressure(VapourVolumeFraction, OxygenVolumeFraction, OxygenUtilization, AirSupplyPressure);
end

== matlab function EVCS_model_v2/supervisor/MATLAB Function ==
  data: P_EV_demand input; en_PV output; P_PV_avail input; SOC_BESS input; V_bus input; t input; mode_cmd input; en_BESS_dis output; en_BESS_chg output; en_FC output; en_GRID output; mode output; dbg_state output; dbg_src_idx output; P parameter
function [en_PV, en_BESS_dis, en_BESS_chg, en_FC, en_GRID, mode, ...
          dbg_state, dbg_src_idx] = ...
   evcs_supervisor(P_EV_demand, P_PV_avail, SOC_BESS, ...
                   V_bus, t, mode_cmd, P)
%#codegen
% EVCS_SUPERVISOR  Mutually-exclusive source selector for the EV charger
%                  + BESS-from-solar charging arbitration.
%
% Drop-in code for a Simulink "MATLAB Function" block.
%
% NOTE: This version assumes there is NO electrolyser / H2 tank in the
%       Simscape model.  The Fuel Cell Stack is modelled as an
%       always-available backup generator, with only ramp-rate /
%       minimum-ON-time protection enforced by the supervisor.
% --------------------------------------------------------------------
% INPUTS
%   P_EV_demand : W    instantaneous EV charging power demand
%   P_PV_avail  : W    available PV power (after MPPT)
%   SOC_BESS    : %    BESS state of charge (0..100)
%   V_bus       : V    measured DC-bus voltage
%   t           : s    simulation time
%   mode_cmd    : int  external override (from RL/RBC):
%                       0 = AUTO  (let supervisor decide)
%                       1 = force PV   2 = BESS  3 = FC  4 = GRID
%                       5 = PV->BESS charging (no EV supply)
%   P           : struct of all parameters (from evcs_params.m)
%
% OUTPUTS  (all ENABLE pins are 0 / 1)
%   en_PV       : enable PV boost converter PWM
%   en_BESS_dis : enable BESS converter in DISCHARGE direction
%   en_BESS_chg : enable BESS converter in CHARGE direction
%   en_FC       : enable FC boost converter PWM
%   en_GRID     : enable VSC PWM (grid rectifier)
%   mode        : actual mode taken this step (0..5)
%
% INVARIANTS
%   * Exactly ONE of {en_PV, en_BESS_dis, en_FC, en_GRID} is high
%     whenever an EV is being supplied (modes 1..4).
%   * en_BESS_chg can be high ONLY in mode 1 (PV+surplus) or mode 5.
%   * en_BESS_chg and en_BESS_dis are NEVER both 1.
% --------------------------------------------------------------------

%% --- persistent state for hysteresis / dwell / FC min-ON ----------
persistent last_mode last_switch_t fc_started_at
if isempty(last_mode)
    last_mode      = int32(0);
    last_switch_t  = -1e9;
    fc_started_at  = -1e9;
end

%% --- 1. compute the "ideal" mode this step --------------------------
ideal = int32(0);

if mode_cmd ~= 0
    % external override (from your RL agent / RBC)
    ideal = int32(mode_cmd);
else
    % ---- automatic priority logic ---------------------------------
    pv_ok    = P_PV_avail >= P.SUP.PV_min;
    bess_dis = SOC_BESS  >  P.SUP.SOC_low;
    bess_chg = SOC_BESS  <  P.SUP.SOC_high;
    fc_ok    = (P.SUP.FC_enable == 1);   % no fuel-tracking; just an enable

    if P_EV_demand < 100        % no EV plugged in
        if pv_ok && bess_chg
            ideal = int32(5);   % PV --> BESS only
        else
            ideal = int32(0);   % everything off
        end
    else
        % EV is charging -- pick the cheapest / greenest source
        if pv_ok && P_PV_avail >= P_EV_demand
            ideal = int32(1);   % PV alone (surplus may also charge BESS)
        elseif bess_dis
            ideal = int32(2);   % BESS
        elseif fc_ok
            ideal = int32(3);   % FC
        else
            ideal = int32(4);   % grid (last resort)
        end
    end
end

%% --- 2. enforce minimum dwell time ---------------------------------
if (t - last_switch_t) < P.SUP.dwell_time && last_mode ~= 0
    chosen = last_mode;
else
    chosen = ideal;
    if chosen ~= last_mode
        last_switch_t = t;
        last_mode     = chosen;
        if chosen == 3
            fc_started_at = t;     % stamp when FC came online
        end
    end
end

%% --- 3. enforce FC minimum ON-time (membrane / thermal safety) ----
% If we are trying to leave FC mode (3) before t_minON has elapsed,
% stay in FC unless the EV is no longer connected.
if last_mode == 3 && chosen ~= 3 && (t - fc_started_at) < P.FC.t_minON
    if P_EV_demand >= 100
        chosen    = int32(3);
        last_mode = chosen;
    end
end

%% --- 4. translate mode --> enable signals --------------------------
en_PV       = uint8(0);
en_BESS_dis = uint8(0);
en_BESS_chg = uint8(0);
en_FC       = uint8(0);
en_GRID     = uint8(0);

switch chosen
    case 1   % PV supplies EV
        en_PV       = uint8(1);
        if (P_PV_avail - P_EV_demand) >= P.SUP.PV_surplus && ...
                SOC_BESS < P.SUP.SOC_high
            en_BESS_chg = uint8(1);   % use surplus to charge BESS
        end
    case 2
        en_BESS_dis = uint8(1);
    case 3
        en_FC       = uint8(1);
    case 4
        en_GRID     = uint8(1);
    case 5   % PV charges BESS, no EV supply
        en_PV       = uint8(1);
        en_BESS_chg = uint8(1);
    otherwise
        % all off
end

%% --- 5. final safety clamp (defence in depth) ----------------------
if en_BESS_dis == 1 && en_BESS_chg == 1
    en_BESS_dis = uint8(0);
    en_BESS_chg = uint8(0);
end

nsupply = double(en_PV) + double(en_BESS_dis) + ...
          double(en_FC) + double(en_GRID);
if nsupply > 1
    en_PV = uint8(0); en_BESS_dis = uint8(0);
    en_FC = uint8(0); en_GRID = uint8(1);
end

%% --- diagnostics ----------------------------------------------------
mode        = int32(chosen);
dbg_state   = [SOC_BESS, V_bus, P_PV_avail, P_EV_demand];
dbg_src_idx = double(chosen);

end

== matlab function EVCS_model_v2/Fuel Cell Stack/Model/Continuous//Detailed/Subsystem1/MATLAB Function12 ==
  data: FuelUtilization input; HydrogenPartialPressure output; FuelVolumeFraction input; FuelSupplyPressure input
function HydrogenPartialPressure = calculateHydrogenPartialPressure(FuelUtilization, FuelVolumeFraction, FuelSupplyPressure)
    % Function to calculate hydrogen partial pressure
    % Copyright 2024 The MathWorks, Inc.
    
    HydrogenPartialPressure = calculatePartialPressure(FuelUtilization, FuelVolumeFraction, FuelSupplyPressure);
end

== matlab function EVCS_model_v2/Fuel Cell Stack/Model/Continuous//Detailed/Subsystem1/MATLAB Function16 ==
  data: HydrogenPartialPressure input; ExchangeCurrentCalculated output; OxygenPartialPressure input; ActivationEnergy input; Temperature input
function ExchangeCurrentCalculated= calculateExchangeCurrent(HydrogenPartialPressure,OxygenPartialPressure,ActivationEnergy,Temperature)
    % Function to calculate Exchange Current Derived
    % Copyright 2024 The MathWorks, Inc.    
    
    F = 96485; % Faraday constant : (A*s/mol)
    k = 1.38e-23; % Boltzmann's constant : (J/K)
    R = 8.3145; % Ideal gas constant : (J/mol*K)
    h = 6.626e-34; % Planck's constant : (J*s)

    ExchangeCurrentCalculated = (2*F*k*(1e5)*(HydrogenPartialPressure + OxygenPartialPressure)/(R*h))*exp(-ActivationEnergy/(R*Temperature));
end

== matlab function EVCS_model_v2/Fuel Cell Stack/Model/Continuous//Detailed/Subsystem1/MATLAB Function18 ==
  data: VoltageUndershoot input; NernstModifierK output; OpenCircuitPotential input; NominalNernst input; MaximumOxygenUtilization input; NominalOxygenUtilization input; NernstModifierKc output; NumberCells input
function [NernstModifierK, NernstModifierKc] = calculateNernstModifiers(VoltageUndershoot, OpenCircuitPotential, NominalNernst, MaximumOxygenUtilization, NominalOxygenUtilization, NumberCells)
    
% Copyright 2024 The MathWorks, Inc.

    [NernstModifierK, NernstModifierKc] = calculateNernstModifiers(VoltageUndershoot, OpenCircuitPotential, NominalNernst, MaximumOxygenUtilization, NominalOxygenUtilization, NumberCells);

end

== matlab function EVCS_model_v2/Fuel Cell Stack/Model/Continuous//Detailed/Subsystem1/MATLAB Function4 ==
  data: Temperature input; FuelUtilization output; Current input; FuelSupplyPressure input; FuelVolumetricFlowRate input; FuelVolumeFraction input; NumberCells input
function FuelUtilization = calculateFuelUtilization(Temperature, Current, FuelSupplyPressure, FuelVolumetricFlowRate, FuelVolumeFraction, NumberCells)
    % Function to calculate oxygen utilization based on the given formula
    % Copyright 2024 The MathWorks, Inc.

    % Constants
    NumberElectrons = 2;
    FuelUtilization = calculateUtilization(Temperature, Current, FuelSupplyPressure, FuelVolumetricFlowRate, FuelVolumeFraction, NumberElectrons, NumberCells);
end

== matlab function EVCS_model_v2/Fuel Cell Stack/Model/Continuous//Detailed/Subsystem1/MATLAB Function5 ==
  data: Temperature input; TafelSlope output; ChargeTransferCoefficient input
function TafelSlope = calculateTafelSlope(Temperature,ChargeTransferCoefficient)

    % Inputs
    % Temperature : (K)
    % ChargeTransferCoefficient : (1)
    % Output
    % ActivationEnergyBarrier : (J)
    % Constants
    F = 96485.33212; % Faraday's constant (C/mol)
    R = 8.3144621; % Universal gas constant (J/(mol*K))
    NumberElectrons = 2;

    % Calculation
    TafelSlope = (R*Temperature)/(NumberElectrons*ChargeTransferCoefficient*F);

== matlab function EVCS_model_v2/Fuel Cell Stack/Model/Continuous//Detailed/Subsystem1/MATLAB Function6 ==
  data: OxygenUtilization input; OxygenPartialPressure output; OxygenVolumeFraction input; AirSupplyPressure input
function OxygenPartialPressure = calculateOxygenPartialPressure(OxygenUtilization, OxygenVolumeFraction, AirSupplyPressure)
    % Function to calculate hydrogen partial pressure
    % Copyright 2024 The MathWorks, Inc.
    
    OxygenPartialPressure = calculatePartialPressure(OxygenUtilization, OxygenVolumeFraction, AirSupplyPressure);
end
